simulink model "test1"  (Simulink 9.2)
settings: Solver=ode45  StartTime=0.0  StopTime=10.0  MaxStep=1e-3  RelTol=1e-6
settings Model: Creator=jinwooro  LastModifiedBy=jinwooro
settings DataIOCC: LimitDataPoints=off  SaveFormat=Dataset  SignalLoggingSaveFormat=Dataset
settings OptimizationCC: LifeSpan=auto
settings DebuggingCC: UnderspecifiedInitializationDetection=Simplified  MergeDetectMultiDrivingBlocksExec=error  FcnCallInpInsideContextMsg=error  StateNameClashWarn=none  SFUnexpectedBacktrackingDiag=error  SFNoUnconditionalDefaultTransitionDiag=error  SFExecutionAtInitializationDiag=warning
settings HardwareCC: ProdBitPerPointer=64  ProdBitPerSizeT=64  ProdBitPerPtrDiffT=64  ProdLargestAtomicFloat=Float  ProdIntDivRoundTo=Zero  ProdEndianess=LittleEndian  ProdWordSize=64  ProdHWDeviceType=Intel->x86-64 (Windows64)
settings ModelReferenceCC: PropagateSignalLabelsOutOfModel=on
settings SFSimCC: SimUseLocalCustomCode=on
settings RTWCC: RTWUseLocalCustomCode=on
settings CodeAppCC: StateflowObjectComments=off
settings GRTTargetCC: TargetLangStandard=C99 (ISO)  GeneratePreprocessorConditionals=Use local settings  CombineOutputUpdateFcns=on  GRTInterface=off
settings ConfigComp: CovMetricSettings=dwe  CovHtmlReporting=off  CovSaveCumulativeToWorkspaceVar=off  CovSaveSingleToWorkspaceVar=off  CovExternalEMLEnable=on

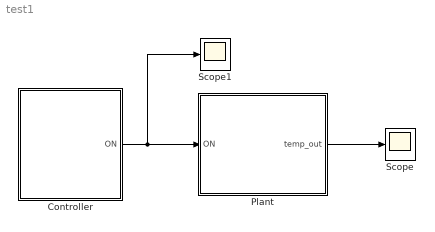
== system test1 ==
  Controller : Stateflow chart  TreatAsAtomicUnit=on
  Plant : Stateflow chart  TreatAsAtomicUnit=on
  Scope : Scope
  Scope1 : Scope
  wires:
  Plant/1(temp_out) -> Scope/1
  Controller/1(ON) -> Scope1/1, Plant/1(ON)

== stateflow chart Controller ==
  settings: updateMethod=CONTINUOUS
  state Idle
    du:
    Time_dot = 1;
    ON = 0;
  state Activated
    du:
    Time_dot = 1;
    ON = 1;
  (default) -> Idle : {
      | Time = 0;
      | }
  Idle -> Activated : [ Time >= 5]
  data: Time local double; ON output double
  data Time settings: updateMethod=SF_CONTINUOUS_TIME_DATA

== stateflow chart Plant ==
  settings: updateMethod=CONTINUOUS
  state Q1
    du:
    temp_dot = 0;
    temp_out = temp;
  state Q2
    du:
    temp_dot = temp * 2;
    temp_out = temp;
  state Q3
    du:
    temp_dot = 0;
    temp_out = temp;
  (default) -> Q1 : {
      | temp = 10;
      | }
  Q1 -> Q2 : [ON == 1]
  Q2 -> Q3 : [temp >= 50]
      | {
      | temp = 0;
      | }
  data: temp local double; temp_out output double; ON input double
  data temp settings: updateMethod=SF_CONTINUOUS_TIME_DATA
